simulink model "FULL_LINK"  (R2021b)
settings: Solver=VariableStepAuto  StartTime=0.0  StopTime=0.04  RelTol=1e-3
undefined symbols (not defined in the file): fcarrier
libraries: fl_lib x21, nesl_utility x7, dspsrcs4 x5, dspswit3 x4, ee_lib x3, dsparch4 x2, simulink x1, hdlsllib x1
settings Model: DataTypeOverride=Off  Creator=hp  LastModifiedBy=caccolillo
settings SolverCC: AlgebraicLoopSolver=TrustRegion  AutoInsertRateTranBlk=on
settings DataIOCC: ReturnWorkspaceOutputs=off
settings OptimizationCC: BlockReduction=off  ConditionallyExecuteInputs=off  DefaultParameterBehavior=Inlined  InheritOutputTypeSmallerThanSingle=on
settings DebuggingCC: AlgebraicLoopMsg=error  SingleTaskRateTransMsg=error  SFMachineParentedDataDiag=warning  ArithmeticOperatorsInVariantConditions=warning
settings HardwareCC: ProdBitPerPointer=32  ProdBitPerSizeT=32  ProdBitPerPtrDiffT=32  ProdLargestAtomicFloat=None  ProdIntDivRoundTo=Undefined  ProdEndianess=Unspecified  ProdWordSize=32  ProdHWDeviceType=ASIC/FPGA->ASIC/FPGA  TargetBitPerLong=64  TargetBitPerPointer=64  TargetBitPerSizeT=64  TargetBitPerPtrDiffT=64  TargetLongLongMode=on  TargetIntDivRoundTo=Zero  TargetEndianess=LittleEndian  TargetWordSize=64  TargetHWDeviceType=Custom Processor->MATLAB Host Computer  ProdEqTarget=off
settings SFSimCC: SimUseLocalCustomCode=off  CustomCodeUndefinedFunction=UseInterfaceOnly
settings RTWCC: RTWUseLocalCustomCode=off

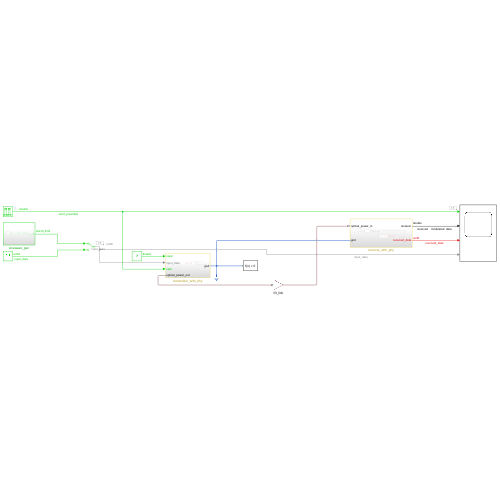
[thumbnail: Simulink's stored preview of the top-level diagram]
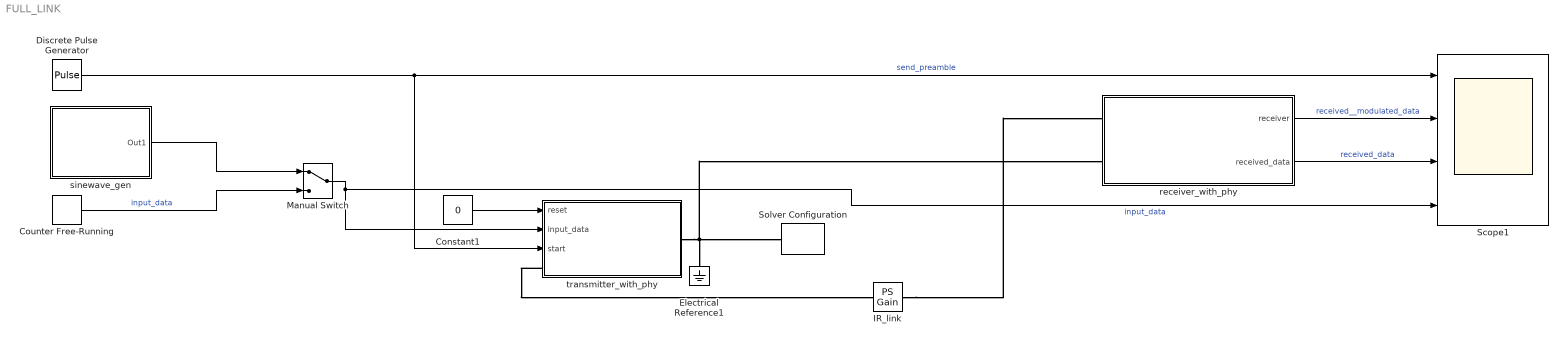
== system FULL_LINK ==
  Constant1 : Constant  Value=0  OutDataTypeStr=double  SampleTime=4/fcarrier
  Counter Free-Running : simulink/Sources/Counter Free-Running  NumBits=8  tsamp=4/fcarrier
  Discrete Pulse Generator : DiscretePulseGenerator  Period=20000  PhaseDelay=80  SampleTime=4/fcarrier
  Electrical Reference1 : fl_lib/Electrical/Electrical Elements/Electrical Reference
  IR_link : fl_lib/Physical Signals/Functions/PS Gain  gain=1e4 1/m^2
  Manual Switch : ManualSwitch
  Scope1 : Scope  NumInputPorts=4
  Solver Configuration : nesl_utility/Solver Configuration  PhysicalDomain=network_engine_domain  SubClassName=solver  LeftPortType=input  RightPortType=generic  Tones=[]  Harmonics=[]  SimulateNoise=off  Profile=off  UseLocalSampling=off  EnableSwitchedLinearOptims=on  FrequencyDomain=off  UseCCode=off  RelTol=0.001  AbsTol=1e-06  MinStep=1e-09  ToWorkspace=off  RevertToSquareIcSolve=off  NumHomotopyIterations=100  PhasorMode=off  PhasorModeNumHarmonics=1  DoDC=off  ResidualTolerance=1e-09  UseLocalSolver=off  LocalSolverChoice=NE_BACKWARD_EULER_ADVANCER  LocalSolverSampleTime=0.001  DoFixedCost=off  MaxNonlinIter=3  MaxModeIter=2  ComputeImpulses=off  ImpulseIterations=2  LinearAlgebra=auto  EquationFormulation=NE_TIME_EF  DelaysMemoryBudget=1024  AutomaticFiltering=on  FilteringTimeConstant=0.001  PartitionStorageMethod=AS_NEEDED  PartitionMemoryBudget=1024  PartitionMethod=ROBUST
      settings: SourceProductBaseCode=PW,SS
  receiver_with_phy : Subsystem
  sinewave_gen : Subsystem
  transmitter_with_phy : Subsystem
  wires:
  Discrete Pulse Generator/1 -> transmitter_with_phy/3(start), Scope1/1  "send_preamble"
  Manual Switch/1 -> transmitter_with_phy/2(input_data), Scope1/4  "input_data"
  Counter Free-Running/1 -> Manual Switch/2  "input_data"
  Constant1/1 -> transmitter_with_phy/1(reset)
  receiver_with_phy/2(received_data) -> Scope1/3  "received_data"
  receiver_with_phy/1(receiver) -> Scope1/2  "received__modulated_data"
  sinewave_gen/1(Out1) -> Manual Switch/1
  connections:
  transmitter_with_phy/RConn1 -- receiver_with_phy/LConn2 -- Solver Configuration/RConn1 -- Electrical Reference1/LConn1
  transmitter_with_phy/LConn1 -- IR_link/LConn1
  IR_link/RConn1 -- receiver_with_phy/LConn1

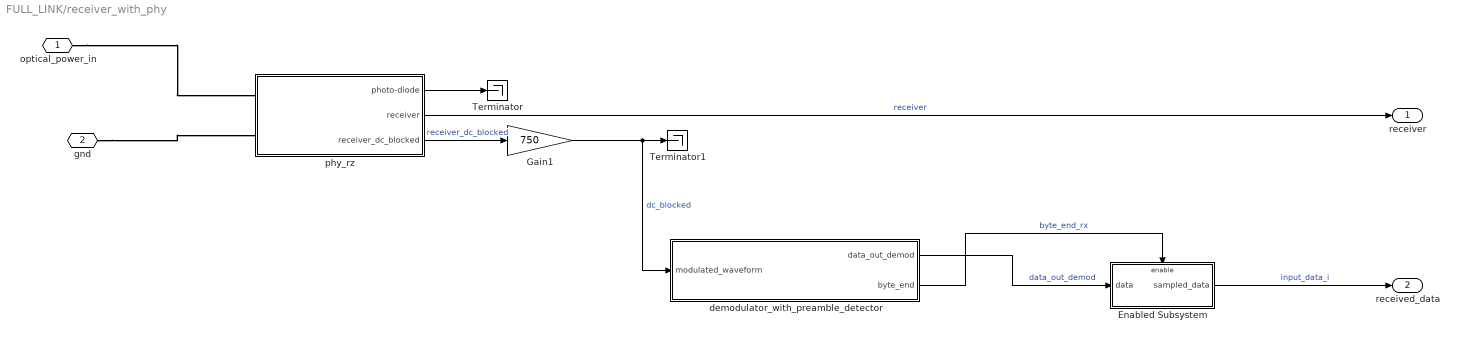
== system FULL_LINK/receiver_with_phy ==
  Enabled Subsystem : Subsystem  TreatAsAtomicUnit=on
  Gain1 : Gain  Gain=750
  Terminator : Terminator
  Terminator1 : Terminator
  demodulator_with_preamble_detector : Subsystem
  phy_rz : Subsystem
  optical_power_in : PMIOPort  Side=Left
  gnd : PMIOPort  Port=2  Side=Left
  receiver : Outport
  received_data : Outport  Port=2
  wires:
  phy_rz/3(receiver_dc_blocked) -> Gain1/1  "receiver_dc_blocked"
  phy_rz/1(photo-diode) -> Terminator/1
  Gain1/1 -> Terminator1/1, demodulator_with_preamble_detector/1(modulated_waveform)  "dc_blocked"
  demodulator_with_preamble_detector/2(byte_end) -> Enabled Subsystem/Enable  "byte_end_rx"
  phy_rz/2(receiver) -> receiver/1  "receiver"
  Enabled Subsystem/1(sampled_data) -> received_data/1  "input_data_i"
  demodulator_with_preamble_detector/1(data_out_demod) -> Enabled Subsystem/1(data)  "data_out_demod"
  connections:
  gnd/RConn1 -- phy_rz/LConn2
  optical_power_in/RConn1 -- phy_rz/LConn1

== system FULL_LINK/sinewave_gen ==
  Add Constant : Bias  Bias=128
  Data Type Conversion1 : DataTypeConversion  OutDataTypeStr=uint8
  Gain2 : Gain  Gain=1/4
  Sine Wave2 : dspsrcs4/Sine Wave  Amplitude=128  Frequency=fcarrier/150  Phase=0  SampleMode=Discrete  OutComplex=Real  CompMethod=Trigonometric fcn  TableSize=Speed  SampleTime=4/fcarrier  SamplesPerFrame=1  ResetState=Restart at time zero  OutputFrames=off  dataType=double  wordLen=16  udDataType=sfix(16)  fracBitsMode=Best precision  numFracBits=15  OutDataTypeStr=double  LastOutDataTypeStr=double
  Out1 : Outport
  wires:
  Sine Wave2/1 -> Data Type Conversion1/1
  Gain2/1 -> Out1/1
  Data Type Conversion1/1 -> Add Constant/1
  Add Constant/1 -> Gain2/1

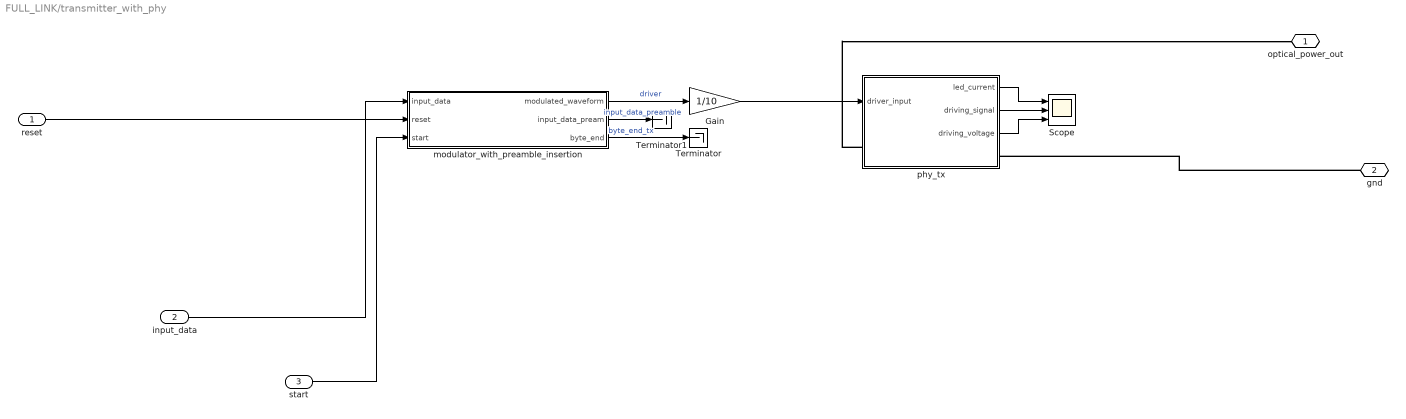
== system FULL_LINK/transmitter_with_phy ==
  reset : Inport
  input_data : Inport  Port=2
  start : Inport  Port=3
  Gain : Gain  Gain=1/10
  Scope : Scope  NumInputPorts=3
  Terminator : Terminator
  Terminator1 : Terminator
  modulator_with_preamble_insertion : Subsystem
  phy_tx : Subsystem
  optical_power_out : PMIOPort  Side=Left
  gnd : PMIOPort  Port=2  Side=Right
  wires:
  phy_tx/1(led_current) -> Scope/1
  Gain/1 -> phy_tx/1(driver_input)
  modulator_with_preamble_insertion/2(input_data_pream) -> Terminator1/1  "input_data_preamble"
  modulator_with_preamble_insertion/3(byte_end) -> Terminator/1  "byte_end_tx"
  start/1 -> modulator_with_preamble_insertion/3(start)
  phy_tx/2(driving_signal) -> Scope/2
  modulator_with_preamble_insertion/1(modulated_waveform) -> Gain/1  "driver"
  input_data/1 -> modulator_with_preamble_insertion/1(input_data)
  reset/1 -> modulator_with_preamble_insertion/2(reset)
  phy_tx/3(driving_voltage) -> Scope/3
  connections:
  gnd/RConn1 -- phy_tx/RConn1
  phy_tx/LConn1 -- optical_power_out/RConn1

== system FULL_LINK/receiver_with_phy/Enabled Subsystem ==
  data : Inport
  Enable : EnablePort
  sampled_data : Outport  InitialOutput=0
  wires:
  data/1 -> sampled_data/1

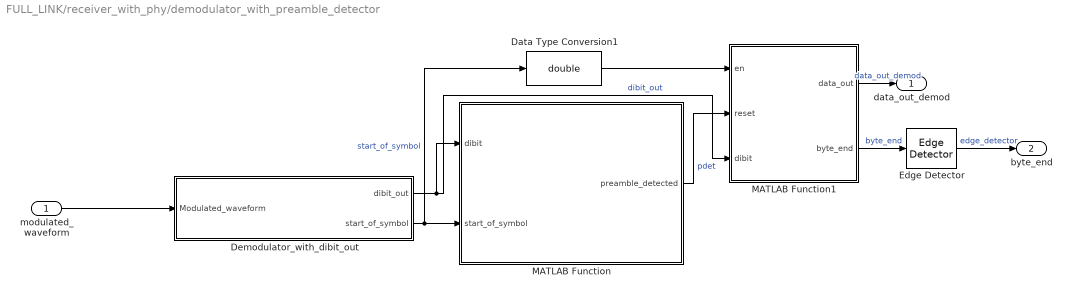
== system FULL_LINK/receiver_with_phy/demodulator_with_preamble_detector ==
  modulated_waveform : Inport
  Data Type Conversion1 : DataTypeConversion  OutDataTypeStr=double
  Demodulator_with_dibit_out : Subsystem
  Edge Detector : dspswit3/Edge Detector  InputProcessing=Columns as channels (frame based)
      settings: SourceProductBaseCode=DS
  MATLAB Function : MATLAB Function  TreatAsAtomicUnit=on
  MATLAB Function1 : MATLAB Function  TreatAsAtomicUnit=on
  data_out_demod : Outport
  byte_end : Outport  Port=2
  wires:
  Demodulator_with_dibit_out/1(dibit_out) -> MATLAB Function/1(dibit), MATLAB Function1/3(dibit)  "dibit_out"
  Demodulator_with_dibit_out/2(start_of_symbol) -> MATLAB Function/2(start_of_symbol), Data Type Conversion1/1  "start_of_symbol"
  Edge Detector/1 -> byte_end/1  "edge_detector"
  modulated_waveform/1 -> Demodulator_with_dibit_out/1(Modulated_waveform)
  MATLAB Function/1(preamble_detected) -> MATLAB Function1/2(reset)  "pdet"
  Data Type Conversion1/1 -> MATLAB Function1/1(en)
  MATLAB Function1/1(data_out) -> data_out_demod/1  "data_out_demod"
  MATLAB Function1/2(byte_end) -> Edge Detector/1  "byte_end"

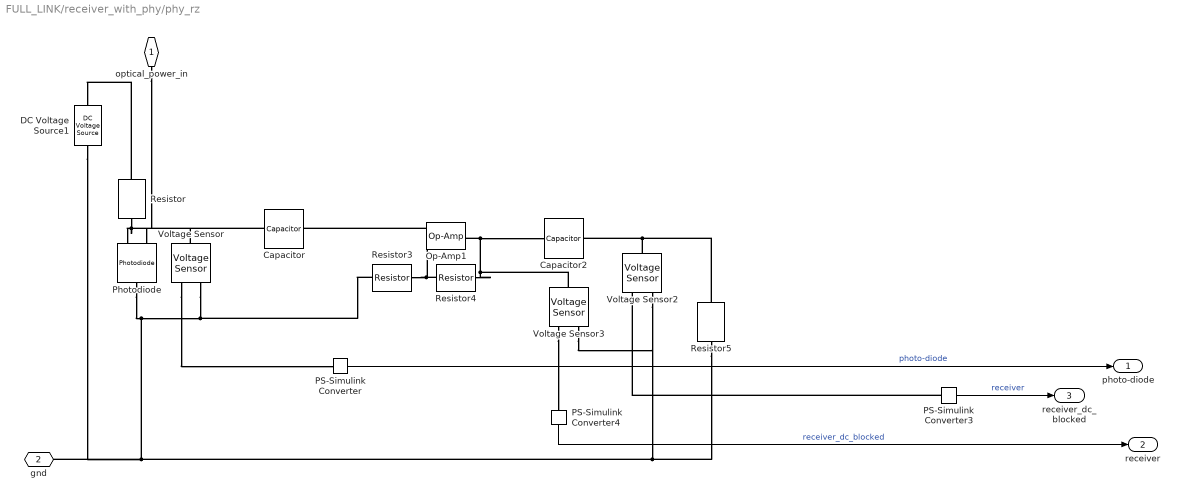
== system FULL_LINK/receiver_with_phy/phy_rz ==
  Capacitor : fl_lib/Electrical/Electrical Elements/Capacitor  c=10 uF  r=0 Ohm  g=0 1/Ohm  i_specify=off  i_priority=None  i=0 A  i_nominal_specify=off  i_nominal_unit=A  i_nominal_value=1  v_specify=off  v_priority=None  v=0 V  v_nominal_specify=off  v_nominal_unit=V  v_nominal_value=1  vc_specify=off  vc_priority=High  vc=0 V  vc_nominal_specify=off  vc_nominal_unit=V  vc_nominal_value=1
  Capacitor2 : fl_lib/Electrical/Electrical Elements/Capacitor  c=1 uF  r=0 Ohm  g=0 1/Ohm  i_specify=off  i_priority=None  i=0 A  i_nominal_specify=off  i_nominal_unit=A  i_nominal_value=1  v_specify=off  v_priority=None  v=0 V  v_nominal_specify=off  v_nominal_unit=V  v_nominal_value=1  vc_specify=off  vc_priority=High  vc=0 V  vc_nominal_specify=off  vc_nominal_unit=V  vc_nominal_value=1
  DC Voltage Source1 : fl_lib/Electrical/Electrical Sources/DC Voltage Source  v0=5 V
  Op-Amp1 : fl_lib/Electrical/Electrical Elements/Op-Amp  outI_specify=off  outI_priority=None  outI=0 A  outI_nominal_specify=off  outI_nominal_unit=A  outI_nominal_value=1
  PS-Simulink Converter : nesl_utility/PS-Simulink Converter  PhysicalDomain=network_engine_domain  SubClassName=ps_output  LeftPortType=input  RightPortType=output  PseudoPeriodic=off  Frequencies=[]  Unit=inherit  AffineConversion=off
      settings: SourceProductBaseCode=PW,SS
  PS-Simulink Converter3 : nesl_utility/PS-Simulink Converter  PhysicalDomain=network_engine_domain  SubClassName=ps_output  LeftPortType=input  RightPortType=output  PseudoPeriodic=off  Frequencies=[]  Unit=inherit  AffineConversion=off
      settings: SourceProductBaseCode=PW,SS
  PS-Simulink Converter4 : nesl_utility/PS-Simulink Converter  PhysicalDomain=network_engine_domain  SubClassName=ps_output  LeftPortType=input  RightPortType=output  PseudoPeriodic=off  Frequencies=[]  Unit=inherit  AffineConversion=off
      settings: SourceProductBaseCode=PW,SS
  Photodiode : ee_lib/Sensors & Transducers/Photodiode  prmFlux=1  Imeas=25 uA  FluxD=5 W/m^2  G=5e-6 A*m^2/W  prmExp=1  I2=0.1 A  V2=1.3 V  IS=5e-9 A  ec=3  RS=0.1 Ohm  Tmeas=25 degC  C_param=1  CJ=60 pF  CJ0=60 pF  VJ=1 V  Mgrad=0.5  Vvec=[.1, 10, 100] V  Cvec=[45, 3, 6] pF  FC=0.5  T_param=1  IS_T2=2.5e-7 A  I1_T2=0.07 A  V1_T2=1.3 V  Tmeas2=125 degC  EG_param=1  EG=1.11 eV  XTI_param=1  XTI=3  Tdevice=25 degC  i_capacitor_specify=off  i_capacitor_priority=High  i_capacitor=0 A  i_capacitor_nominal_specify=off  i_capacitor_nominal_unit=A  i_capacitor_nominal_value=1  v_capacitor_specify=off  v_capacitor_priority=None  v_capacitor=0 V  v_capacitor_nominal_specify=off  v_capacitor_nominal_unit=V  v_capacitor_nominal_value=1  thermal_network_parameterization=ee.enum.thermalNetworkTopology.junctionCase  Rth=[0, 10] K/W  Rth_Cauer=[1, 3, 10] K/W  Rth_Foster=[4, 6] K/W  thermal_mass_parameterization=ee.enum.thermalNetwork.timeconstant  thermal_mass=[0, 1] J/K  thermal_mass_Cauer=[1.5, 2, 3] J/K  thermal_mass_Foster=[1.5, 3] J/K  thermal_time_constant=[0, 10] s  thermal_time_constant_Cauer=[1, 3, 10] s  thermal_time_constant_Foster=[6, 18] s  thermal_mass_initial_temperatures=[25, 25] degC  thermal_mass_initial_temperatures_Cauer=[25, 25, 25] degC  steadyState_Foster=simscape.enum.onoff.on  Tvec_initial_Foster=[25, 25, 25, 25] degC
      settings: SourceProductBaseCode=PS  InternalSimscapePortConfiguration="{\"Bottom\":[],\"Left\":[{\"id\":\"W\",\"label\":\"W\",\"type\":\"input\"},{\"id\":\"p\",\"label\":\"\",\"type\":\"foundation.electrical.electrical\"}],\"Right\":[{\"id\":\"n\",\"label\":\"\",\"type\":\"foundation.electrical.electrical\"}],\"Top\":[]}"
  Resistor : fl_lib/Electrical/Electrical Elements/Resistor  R=1000 Ohm  i_specify=off  i_priority=None  i=0 A  i_nominal_specify=off  i_nominal_unit=A  i_nominal_value=1  v_specify=off  v_priority=None  v=0 V  v_nominal_specify=off  v_nominal_unit=V  v_nominal_value=1
  Resistor3 : fl_lib/Electrical/Electrical Elements/Resistor  R=1000 Ohm  i_specify=off  i_priority=None  i=0 A  i_nominal_specify=off  i_nominal_unit=A  i_nominal_value=1  v_specify=off  v_priority=None  v=0 V  v_nominal_specify=off  v_nominal_unit=V  v_nominal_value=1
  Resistor4 : fl_lib/Electrical/Electrical Elements/Resistor  R=20000 Ohm  i_specify=off  i_priority=None  i=0 A  i_nominal_specify=off  i_nominal_unit=A  i_nominal_value=1  v_specify=off  v_priority=None  v=0 V  v_nominal_specify=off  v_nominal_unit=V  v_nominal_value=1
  Resistor5 : fl_lib/Electrical/Electrical Elements/Resistor  R=1 kOhm  i_specify=off  i_priority=None  i=5 mA  i_nominal_specify=off  i_nominal_unit=A  i_nominal_value=1  v_specify=off  v_priority=None  v=0 V  v_nominal_specify=off  v_nominal_unit=V  v_nominal_value=1
  Voltage Sensor : fl_lib/Electrical/Electrical Sensors/Voltage Sensor
  Voltage Sensor2 : fl_lib/Electrical/Electrical Sensors/Voltage Sensor
  Voltage Sensor3 : fl_lib/Electrical/Electrical Sensors/Voltage Sensor
  optical_power_in : PMIOPort  Side=Left
  gnd : PMIOPort  Port=2  Side=Left
  photo-diode : Outport
  receiver : Outport  Port=2
  receiver_dc_blocked : Outport  Port=3
  wires:
  PS-Simulink Converter/1 -> photo-diode/1  "photo-diode"
  PS-Simulink Converter4/1 -> receiver/1  "receiver_dc_blocked"
  PS-Simulink Converter3/1 -> receiver_dc_blocked/1  "receiver"
  connections:
  PS-Simulink Converter3/LConn1 -- Voltage Sensor2/RConn1
  Resistor4/LConn1 -- Voltage Sensor3/LConn1 -- Capacitor2/LConn1 -- Op-Amp1/RConn1
  optical_power_in/RConn1 -- Photodiode/LConn1
  Resistor3/LConn1 -- Op-Amp1/LConn2 -- Resistor4/RConn1
  Op-Amp1/LConn1 -- Capacitor/RConn1
  Voltage Sensor3/RConn1 -- PS-Simulink Converter4/LConn1
  Resistor5/LConn1 -- Voltage Sensor2/RConn2 -- Voltage Sensor3/RConn2 -- Photodiode/RConn1 -- Resistor3/RConn1 -- Voltage Sensor/RConn2 -- DC Voltage Source1/RConn1 -- gnd/RConn1
  Voltage Sensor2/LConn1 -- Resistor5/RConn1 -- Capacitor2/RConn1
  Voltage Sensor/RConn1 -- PS-Simulink Converter/LConn1
  Resistor/LConn1 -- DC Voltage Source1/LConn1
  Resistor/RConn1 -- Voltage Sensor/LConn1 -- Capacitor/LConn1 -- Photodiode/LConn2

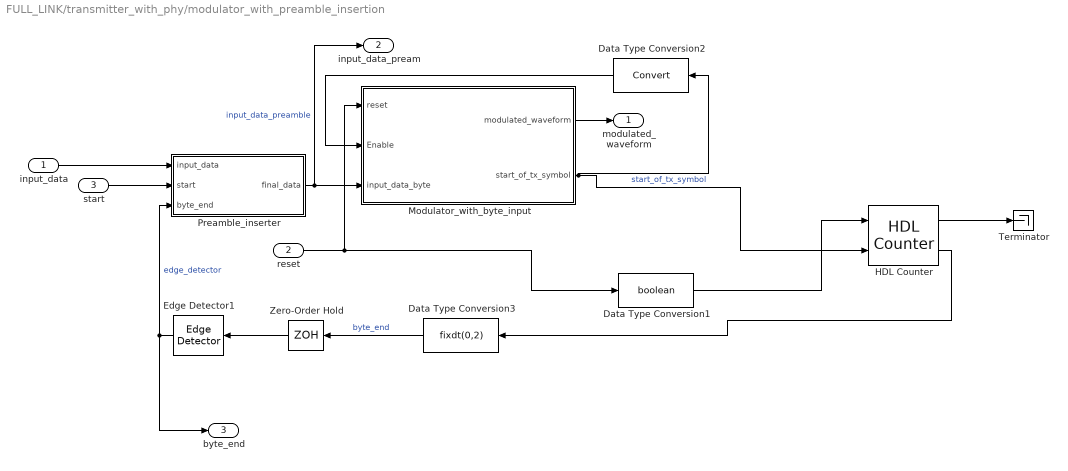
== system FULL_LINK/transmitter_with_phy/modulator_with_preamble_insertion ==
  input_data : Inport
  reset : Inport  Port=2
  start : Inport  Port=3
  Data Type Conversion1 : DataTypeConversion  OutDataTypeStr=boolean
  Data Type Conversion2 : DataTypeConversion
  Data Type Conversion3 : DataTypeConversion  OutMin=[0]  OutMax=[1]  OutDataTypeStr=fixdt(0,2)
  Edge Detector1 : dspswit3/Edge Detector  InputProcessing=Columns as channels (frame based)
      settings: SourceProductBaseCode=DS
  HDL Counter : hdlsllib/Sources/HDL Counter  CountType=Count limited  CountInit=0  CountStep=1  CountMax=7  CountFromType=Initial value  CountFrom=0  CountResetPort=on  CountLoadPort=off  CountEnbPort=on  CountDirPort=off  CountHitOutputPort=on  CountDataType=Unsigned  CountWordLen=8  CountFracLen=0  CountSampTime=1
  Modulator_with_byte_input : Subsystem
  Preamble_inserter : Subsystem
  Terminator : Terminator
  Zero-Order Hold : ZeroOrderHold  SampleTime=-1
  modulated_waveform : Outport
  input_data_pream : Outport  Port=2
  byte_end : Outport  Port=3
  wires:
  reset/1 -> Data Type Conversion1/1, Modulator_with_byte_input/1(reset)
  Modulator_with_byte_input/2(start_of_tx_symbol) -> HDL Counter/2, Data Type Conversion2/1  "start_of_tx_symbol"
  Data Type Conversion2/1 -> Modulator_with_byte_input/2(Enable)
  Modulator_with_byte_input/1(modulated_waveform) -> modulated_waveform/1
  Preamble_inserter/1(final_data) -> Modulator_with_byte_input/3(input_data_byte), input_data_pream/1  "input_data_preamble"
  Data Type Conversion3/1 -> Zero-Order Hold/1  "byte_end"
  HDL Counter/2 -> Data Type Conversion3/1
  start/1 -> Preamble_inserter/2(start)
  input_data/1 -> Preamble_inserter/1(input_data)
  Edge Detector1/1 -> byte_end/1, Preamble_inserter/3(byte_end)  "edge_detector"
  HDL Counter/1 -> Terminator/1
  Data Type Conversion1/1 -> HDL Counter/1
  Zero-Order Hold/1 -> Edge Detector1/1

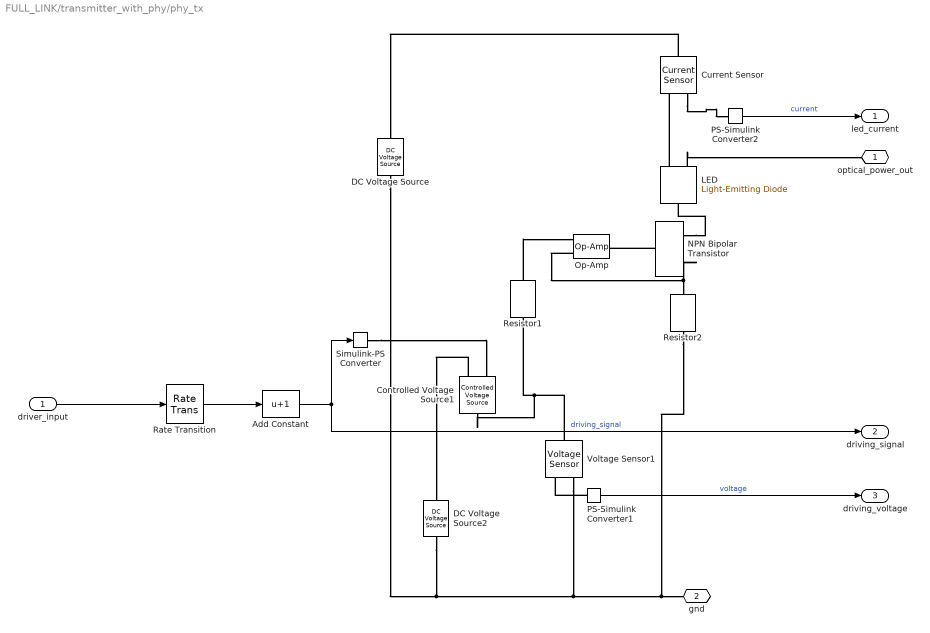
== system FULL_LINK/transmitter_with_phy/phy_tx ==
  driver_input : Inport
  Add Constant : Bias  Bias=1
  Controlled Voltage Source1 : fl_lib/Electrical/Electrical Sources/Controlled Voltage Source
  Current Sensor : fl_lib/Electrical/Electrical Sensors/Current Sensor
  DC Voltage Source : fl_lib/Electrical/Electrical Sources/DC Voltage Source  v0=3 V
  DC Voltage Source2 : fl_lib/Electrical/Electrical Sources/DC Voltage Source  v0=0.1 V
  LED : ee_lib/Sensors & Transducers/Light-Emitting Diode  Gain=0.005 W/A  prmExp=1  I12=[.0017, .003] A  V12=[.9, 1.05] V  IS=5e-5 A  ec=10  RS=0.1 Ohm  Tmeas=25 degC  C_param=1  CJ=20 pF  CJ0=20 pF  VJ=1 V  Mgrad=0.5  Vvec=[.1, 10, 100] V  Cvec=[15, 10, 2] pF  FC=0.5  T_param=1  IS_T2=1.8e-4 A  I1_T2=0.0034 A  V1_T2=1.05 V  Tmeas2=125 degC  EG_param=1  EG=1.11 eV  XTI_param=1  XTI=3  Tdevice=25 degC  i_capacitor_specify=off  i_capacitor_priority=High  i_capacitor=0 A  i_capacitor_nominal_specify=off  i_capacitor_nominal_unit=A  i_capacitor_nominal_value=1  v_capacitor_specify=off  v_capacitor_priority=None  v_capacitor=0 V  v_capacitor_nominal_specify=off  v_capacitor_nominal_unit=V  v_capacitor_nominal_value=1  thermal_network_parameterization=ee.enum.thermalNetworkTopology.junctionCase  Rth=[0, 10] K/W  Rth_Cauer=[1, 3, 10] K/W  Rth_Foster=[4, 6] K/W  thermal_mass_parameterization=ee.enum.thermalNetwork.timeconstant  thermal_mass=[0, 1] J/K  thermal_mass_Cauer=[1.5, 2, 3] J/K  thermal_mass_Foster=[1.5, 3] J/K  thermal_time_constant=[0, 10] s  thermal_time_constant_Cauer=[1, 3, 10] s  thermal_time_constant_Foster=[6, 18] s  thermal_mass_initial_temperatures=[25, 25] degC  thermal_mass_initial_temperatures_Cauer=[25, 25, 25] degC  steadyState_Foster=simscape.enum.onoff.on  Tvec_initial_Foster=[25, 25, 25, 25] degC
      settings: SourceProductBaseCode=PS  InternalSimscapePortConfiguration="{\"Bottom\":[],\"Left\":[{\"id\":\"W\",\"label\":\"W\",\"type\":\"output\"},{\"id\":\"p\",\"label\":\"\",\"type\":\"foundation.electrical.electrical\"}],\"Right\":[{\"id\":\"n\",\"label\":\"\",\"type\":\"foundation.electrical.electrical\"}],\"Top\":[]}"
  NPN Bipolar Transistor : ee_lib/Semiconductors & Converters/NPN Bipolar Transistor  parameterization=1  BF=100  IS=1e-14 A  VAF=200 V  hfe=100  hoe=50e-6 1/Ohm  Ic_h=1 mA  Vce_h=5 V  V1=0.55 V  I1=0.5 mA  BR=1  Tmeas=25 degC  RC=0.01 Ohm  RE=1e-4 Ohm  RB=1 Ohm  C_BC=5 pF  C_BE=5 pF  TF=0 us  TR=0 us  prmDatasheet=1  prmEquCoeff=1  hfe_T2=125  XTB=0  V1_T2=0.45 V  I1_T2=0.5 mA  Tmeas2=125 degC  EG=1.11 eV  XTI=3  TdeviceDatasheet=25 degC  TdeviceEquCoeff=25 degC  ec=1  thermal_network_parameterization=ee.enum.thermalNetworkTopology.junctionCase  Rth=[0, 10] K/W  Rth_Cauer=[1, 3, 10] K/W  Rth_Foster=[4, 6] K/W  thermal_mass_parameterization=ee.enum.thermalNetwork.timeconstant  thermal_mass=[0, 1] J/K  thermal_mass_Cauer=[.1, .3, 1] J/K  thermal_mass_Foster=[1.5, 3] J/K  thermal_time_constant=[0, 10] s  thermal_time_constant_Cauer=[1, 3, 10] s  thermal_time_constant_Foster=[6, 18] s  thermal_mass_initial_temperatures=[25, 25] degC  thermal_mass_initial_temperatures_Cauer=[25, 25, 25] degC  steadyState_Foster=simscape.enum.onoff.on  Tvec_initial_Foster=[25, 25, 25, 25] degC
  Op-Amp : fl_lib/Electrical/Electrical Elements/Op-Amp  outI_specify=off  outI_priority=None  outI=0 A  outI_nominal_specify=off  outI_nominal_unit=A  outI_nominal_value=1
  PS-Simulink Converter1 : nesl_utility/PS-Simulink Converter  PhysicalDomain=network_engine_domain  SubClassName=ps_output  LeftPortType=input  RightPortType=output  PseudoPeriodic=off  Frequencies=[]  Unit=inherit  AffineConversion=off
      settings: SourceProductBaseCode=PW,SS
  PS-Simulink Converter2 : nesl_utility/PS-Simulink Converter  PhysicalDomain=network_engine_domain  SubClassName=ps_output  LeftPortType=input  RightPortType=output  PseudoPeriodic=off  Frequencies=[]  Unit=inherit  AffineConversion=off
      settings: SourceProductBaseCode=PW,SS
  Rate Transition : RateTransition
  Resistor1 : fl_lib/Electrical/Electrical Elements/Resistor  R=500 Ohm  i_specify=off  i_priority=None  i=0 A  i_nominal_specify=off  i_nominal_unit=A  i_nominal_value=1  v_specify=off  v_priority=None  v=0 V  v_nominal_specify=off  v_nominal_unit=V  v_nominal_value=1
  Resistor2 : fl_lib/Electrical/Electrical Elements/Resistor  R=10 Ohm  i_specify=off  i_priority=None  i=0 A  i_nominal_specify=off  i_nominal_unit=A  i_nominal_value=1  v_specify=off  v_priority=None  v=0 V  v_nominal_specify=off  v_nominal_unit=V  v_nominal_value=1
  Simulink-PS Converter : nesl_utility/Simulink-PS Converter  PhysicalDomain=network_engine_domain  SubClassName=ps_input  LeftPortType=input  RightPortType=output  PseudoPeriodic=off  Frequencies=[]  NoiseDistribution=none  NoiseParameters=[]  Unit=1  AffineConversion=off  FilteringAndDerivatives=provide  SimscapeFilterOrder=1  InputFilterTimeConstant=0.001  UdotUserProvided=0
      settings: SourceProductBaseCode=PW,SS
  Voltage Sensor1 : fl_lib/Electrical/Electrical Sensors/Voltage Sensor
  optical_power_out : PMIOPort  Side=Left
  gnd : PMIOPort  Port=2  Side=Right
  led_current : Outport
  driving_signal : Outport  Port=2
  driving_voltage : Outport  Port=3
  wires:
  PS-Simulink Converter2/1 -> led_current/1  "current"
  PS-Simulink Converter1/1 -> driving_voltage/1  "voltage"
  Add Constant/1 -> driving_signal/1, Simulink-PS Converter/1  "driving_signal"
  driver_input/1 -> Rate Transition/1
  Rate Transition/1 -> Add Constant/1
  connections:
  Controlled Voltage Source1/RConn2 -- DC Voltage Source2/LConn1
  Resistor1/RConn1 -- Op-Amp/LConn1
  Current Sensor/LConn1 -- DC Voltage Source/LConn1
  LED/LConn1 -- optical_power_out/RConn1
  Simulink-PS Converter/RConn1 -- Controlled Voltage Source1/RConn1
  DC Voltage Source2/RConn1 -- gnd/RConn1 -- Resistor2/RConn1 -- Voltage Sensor1/RConn2 -- DC Voltage Source/RConn1
  Current Sensor/RConn1 -- PS-Simulink Converter2/LConn1
  NPN Bipolar Transistor/RConn2 -- Op-Amp/LConn2 -- Resistor2/LConn1
  NPN Bipolar Transistor/LConn1 -- Op-Amp/RConn1
  NPN Bipolar Transistor/RConn1 -- LED/RConn1
  PS-Simulink Converter1/LConn1 -- Voltage Sensor1/RConn1
  Controlled Voltage Source1/LConn1 -- Voltage Sensor1/LConn1 -- Resistor1/LConn1
  LED/LConn2 -- Current Sensor/RConn2

== system FULL_LINK/receiver_with_phy/demodulator_with_preamble_detector/Demodulator_with_dibit_out ==
  Modulated_waveform : Inport
  Convert_to_decimal : Subsystem
  Demodulator_with_output_register : Subsystem
  dibit_out : Outport
  start_of_symbol : Outport  Port=2
  wires:
  Demodulator_with_output_register/1(i_demod) -> Convert_to_decimal/2(bit1)
  Demodulator_with_output_register/2(q_demod) -> Convert_to_decimal/1(bit0)
  Convert_to_decimal/1(convert) -> dibit_out/1  "dibit_out"
  Demodulator_with_output_register/3(start_of_symbol) -> start_of_symbol/1
  Modulated_waveform/1 -> Demodulator_with_output_register/1(Modulated_waveform)

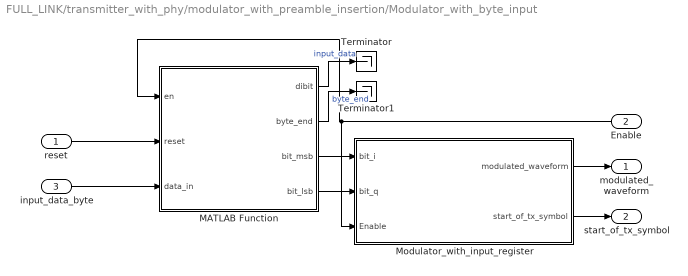
== system FULL_LINK/transmitter_with_phy/modulator_with_preamble_insertion/Modulator_with_byte_input ==
  reset : Inport
  Enable : Inport  Port=2
  input_data_byte : Inport  Port=3
  MATLAB Function : MATLAB Function  TreatAsAtomicUnit=on
  Modulator_with_input_register : Subsystem
  Terminator : Terminator
  Terminator1 : Terminator
  modulated_waveform : Outport
  start_of_tx_symbol : Outport  Port=2
  wires:
  Enable/1 -> MATLAB Function/1(en), Modulator_with_input_register/3(Enable)
  MATLAB Function/2(byte_end) -> Terminator1/1  "byte_end"
  Modulator_with_input_register/2(start_of_tx_symbol) -> start_of_tx_symbol/1
  input_data_byte/1 -> MATLAB Function/3(data_in)
  reset/1 -> MATLAB Function/2(reset)
  MATLAB Function/1(dibit) -> Terminator/1  "input_data"
  MATLAB Function/4(bit_lsb) -> Modulator_with_input_register/2(bit_q)
  Modulator_with_input_register/1(modulated_waveform) -> modulated_waveform/1
  MATLAB Function/3(bit_msb) -> Modulator_with_input_register/1(bit_i)

== system FULL_LINK/transmitter_with_phy/modulator_with_preamble_insertion/Preamble_inserter ==
  input_data : Inport
  start : Inport  Port=2
  byte_end : Inport  Port=3
  Chart : Stateflow chart  TreatAsAtomicUnit=on
      settings: PortSchema="{\"entries\":[{\"content\":{\"sides\":[{\"content\":{\"connectorIds\":[\"In2\"]},\"type\":\"ConnectorPlacement.EquallySpacedRectSide\",\"uuid\":\"c7ea0b9c-d106-4bd1-82e3-4c4e9722273c\"},{\"content\":{\"connectorIds\":[\"Out1\",\"Out2\"],\"side\":\"RIGHT\"},\"type\":\"ConnectorPlacement.EquallySpacedRectSide\",\"uuid\":\"4cc951b6-537b-4e23-ae77-107cf1cb9d20\"},{\"content\":{\"connectorIds\":[\"In1\"],\"side\":\"TOP\"},\"type\":\"ConnectorPlacement.EquallySpacedRectSide\",\"uuid\":\"96187a88-f84a-4d19-a7a7-49870645ca9d\"}]},\"type\":\"ConnectorPlacement.EquallySpacedConnector\",\"uuid\":\"a478a027-a6f7-4a96-ae1b-a22c0dc62afa\"}],\"packageUris\":[\"http://schema.mathworks.com/mf0/Connector/R2020b\"],\"version\":\"1.0\"}"
  Data Type Conversion4 : DataTypeConversion  OutMin=[0]  OutMax=[1]  OutDataTypeStr=double
  Switch : Switch  Criteria=u2 ~= 0  Threshold=1
  final_data : Outport
  wires:
  Switch/1 -> final_data/1  "final_data"
  input_data/1 -> Switch/1
  Data Type Conversion4/1 -> Switch/3
  Chart/2(select_data_preamble) -> Switch/2  "select_data_preamble"
  byte_end/1 -> Chart/1(byte_end)  "byte_end"
  Chart/1(input_data_byte) -> Data Type Conversion4/1  "input_data_byte"
  start/1 -> Chart/2(start)

== system FULL_LINK/receiver_with_phy/demodulator_with_preamble_detector/Demodulator_with_dibit_out/Convert_to_decimal ==
  bit0 : Inport
  bit1 : Inport  Port=2
  Add : Sum
  Gain1 : Gain  Gain=2
  convert : Outport
  wires:
  bit1/1 -> Gain1/1
  bit0/1 -> Add/1
  Add/1 -> convert/1  "convert"
  Gain1/1 -> Add/2

== system FULL_LINK/receiver_with_phy/demodulator_with_preamble_detector/Demodulator_with_dibit_out/Demodulator_with_output_register ==
  Modulated_waveform : Inport
  Demodulator : Subsystem
  Enabled Subsystem2 : Subsystem  TreatAsAtomicUnit=on
  Enabled Subsystem3 : Subsystem  TreatAsAtomicUnit=on
  i_demod : Outport
  q_demod : Outport  Port=2
  start_of_symbol : Outport  Port=3
  wires:
  Demodulator/2(q_demodulator) -> Enabled Subsystem3/1(bit_msb)  "q_demod"
  Demodulator/3(start_of_symbol) -> start_of_symbol/1, Enabled Subsystem3/Enable, Enabled Subsystem2/Enable
  Modulated_waveform/1 -> Demodulator/1(Modulated_waveform)
  Demodulator/1(i_demodulator) -> Enabled Subsystem2/1(bit_msb)  "i_demod"
  Enabled Subsystem2/1(i_data) -> i_demod/1  "i_demod"
  Enabled Subsystem3/1(i_data) -> q_demod/1  "q_demod"

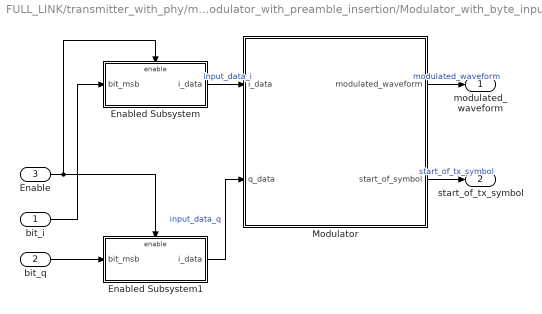
== system FULL_LINK/transmitter_with_phy/modulator_with_preamble_insertion/Modulator_with_byte_input/Modulator_with_input_register ==
  bit_i : Inport
  bit_q : Inport  Port=2
  Enable : Inport  Port=3
  Enabled Subsystem : Subsystem  TreatAsAtomicUnit=on
  Enabled Subsystem1 : Subsystem  TreatAsAtomicUnit=on
  Modulator : Subsystem
  modulated_waveform : Outport
  start_of_tx_symbol : Outport  Port=2
  wires:
  Enabled Subsystem/1(i_data) -> Modulator/1(i_data)  "input_data_i"
  Modulator/2(start_of_symbol) -> start_of_tx_symbol/1  "start_of_tx_symbol"
  bit_q/1 -> Enabled Subsystem1/1(bit_msb)
  bit_i/1 -> Enabled Subsystem/1(bit_msb)
  Enabled Subsystem1/1(i_data) -> Modulator/2(q_data)  "input_data_q"
  Modulator/1(modulated_waveform) -> modulated_waveform/1  "modulated_waveform"
  Enable/1 -> Enabled Subsystem/Enable, Enabled Subsystem1/Enable

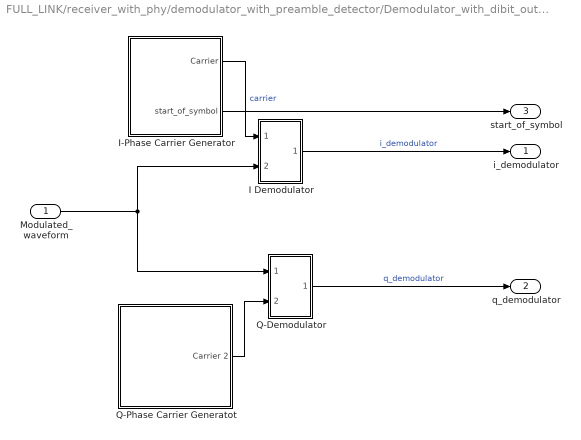
== system FULL_LINK/receiver_with_phy/demodulator_with_preamble_detector/Demodulator_with_dibit_out/Demodulator_with_output_register/Demodulator ==
  Modulated_waveform : Inport
  "I Demodulator " : Subsystem
  "I-Phase Carrier Generator " : Subsystem
  Q-Demodulator : Subsystem
  Q-Phase Carrier Generatot : Subsystem
  i_demodulator : Outport
  q_demodulator : Outport  Port=2
  start_of_symbol : Outport  Port=3
  wires:
  Q-Demodulator/1(Out1) -> q_demodulator/1  "q_demodulator"
  Modulated_waveform/1 -> Q-Demodulator/1(In1), "I Demodulator "/2(In2)
  Q-Phase Carrier Generatot/1("Carrier 2 ") -> Q-Demodulator/2("Carrier 2 ")
  "I Demodulator "/1(Out1) -> i_demodulator/1  "i_demodulator"
  "I-Phase Carrier Generator "/1(Carrier) -> "I Demodulator "/1(Carrier)  "carrier"
  "I-Phase Carrier Generator "/2(start_of_symbol) -> start_of_symbol/1

== system FULL_LINK/receiver_with_phy/demodulator_with_preamble_detector/Demodulator_with_dibit_out/Demodulator_with_output_register/Enabled Subsystem2 ==
  bit_msb : Inport
  Enable : EnablePort
  i_data : Outport  InitialOutput=0
  wires:
  bit_msb/1 -> i_data/1

== system FULL_LINK/receiver_with_phy/demodulator_with_preamble_detector/Demodulator_with_dibit_out/Demodulator_with_output_register/Enabled Subsystem3 ==
  bit_msb : Inport
  Enable : EnablePort
  i_data : Outport  InitialOutput=0
  wires:
  bit_msb/1 -> i_data/1

== system FULL_LINK/transmitter_with_phy/modulator_with_preamble_insertion/Modulator_with_byte_input/Modulator_with_input_register/Enabled Subsystem ==
  bit_msb : Inport
  Enable : EnablePort
  i_data : Outport  InitialOutput=0
  wires:
  bit_msb/1 -> i_data/1

== system FULL_LINK/transmitter_with_phy/modulator_with_preamble_insertion/Modulator_with_byte_input/Modulator_with_input_register/Enabled Subsystem1 ==
  bit_msb : Inport
  Enable : EnablePort
  i_data : Outport  InitialOutput=0
  wires:
  bit_msb/1 -> i_data/1

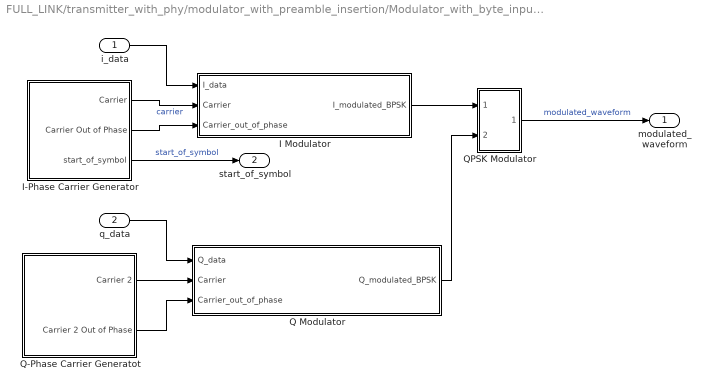
== system FULL_LINK/transmitter_with_phy/modulator_with_preamble_insertion/Modulator_with_byte_input/Modulator_with_input_register/Modulator ==
  i_data : Inport
  q_data : Inport  Port=2
  I Modulator : Subsystem
  "I-Phase Carrier Generator " : Subsystem
  Q Modulator : Subsystem
  Q-Phase Carrier Generatot : Subsystem
  QPSK Modulator : Subsystem
  modulated_waveform : Outport
  start_of_symbol : Outport  Port=2
  wires:
  I Modulator/1(I_modulated_BPSK) -> QPSK Modulator/1(In1)
  q_data/1 -> Q Modulator/1(Q_data)
  i_data/1 -> I Modulator/1(I_data)
  Q Modulator/1("Q_modulated_BPSK ") -> QPSK Modulator/2(In2)
  QPSK Modulator/1(Out1) -> modulated_waveform/1  "modulated_waveform"
  "I-Phase Carrier Generator "/2("Carrier Out of Phase ") -> I Modulator/3(Carrier_out_of_phase)
  Q-Phase Carrier Generatot/1("Carrier 2 ") -> Q Modulator/2(Carrier)
  Q-Phase Carrier Generatot/2(Carrier 2 Out of Phase) -> Q Modulator/3(Carrier_out_of_phase)
  "I-Phase Carrier Generator "/1(Carrier) -> I Modulator/2(Carrier)  "carrier"
  "I-Phase Carrier Generator "/3(start_of_symbol) -> start_of_symbol/1  "start_of_symbol"

== system FULL_LINK/receiver_with_phy/demodulator_with_preamble_detector/Demodulator_with_dibit_out/Demodulator_with_output_register/Demodulator/I Demodulator  ==
  Carrier : Inport
  In2 : Inport  Port=2
  Digital Filter Design : dsparch4/Digital Filter Design  mwdsp_browser_bugfix_var=off
  Product2 : Product
  Relational Operator : RelationalOperator  Operator=<  OutDataTypeStr=boolean  RndMeth=Simplest
  Scope : Scope  NumInputPorts=3
  Zero : Constant  Value=0  SampleTime=1/(100*fcarrier)
  Out1 : Outport  VectorParamsAs1DForOutWhenUnconnected=off
  wires:
  Digital Filter Design/1 -> Scope/3, Relational Operator/1  "filter_out"
  In2/1 -> Product2/2
  Product2/1 -> Scope/2, Digital Filter Design/1  "mixed"
  Zero/1 -> Relational Operator/2
  Relational Operator/1 -> Out1/1
  Carrier/1 -> Scope/1, Product2/1

== system FULL_LINK/receiver_with_phy/demodulator_with_preamble_detector/Demodulator_with_dibit_out/Demodulator_with_output_register/Demodulator/I-Phase Carrier Generator  ==
  Constant1 : Constant  Value=0  OutDataTypeStr=int8  SampleTime=1/(100*fcarrier)
  Data Type Conversion : DataTypeConversion  OutDataTypeStr=int8
  Edge Detector : dspswit3/Edge Detector  InputProcessing=Columns as channels (frame based)
      settings: SourceProductBaseCode=DS
  Equal : RelationalOperator  Operator=>  OutDataTypeStr=boolean  RndMeth=Simplest
  Scope : Scope  NumInputPorts=4
  Sine Wave1 : dspsrcs4/Sine Wave  Amplitude=1  Frequency=fcarrier  Phase=0  SampleMode=Discrete  OutComplex=Real  CompMethod=Trigonometric fcn  TableSize=Speed  SampleTime=1/(100*fcarrier)  SamplesPerFrame=1  ResetState=Restart at time zero  OutputFrames=off  dataType=double  wordLen=16  udDataType=sfix(16)  fracBitsMode=Best precision  numFracBits=15  OutDataTypeStr=double  LastOutDataTypeStr=double
  Carrier : Outport  VectorParamsAs1DForOutWhenUnconnected=off
  start_of_symbol : Outport  Port=2
  wires:
  Constant1/1 -> Equal/1
  Equal/1 -> Scope/2, Edge Detector/1  "start_of_symbol"
  Data Type Conversion/1 -> Scope/1, Equal/2
  Edge Detector/1 -> Scope/4, start_of_symbol/1  "edge_detector"
  Sine Wave1/1 -> Data Type Conversion/1, Scope/3, Carrier/1  "sine"

== system FULL_LINK/receiver_with_phy/demodulator_with_preamble_detector/Demodulator_with_dibit_out/Demodulator_with_output_register/Demodulator/Q-Demodulator ==
  In1 : Inport
  "Carrier 2 " : Inport  Port=2
  Digital Filter Design1 : dsparch4/Digital Filter Design  mwdsp_browser_bugfix_var=off
  Product3 : Product
  Relational Operator1 : RelationalOperator  Operator=<  OutDataTypeStr=boolean  RndMeth=Simplest
  Zero1 : Constant  Value=0  SampleTime=1/(100*fcarrier)
  Out1 : Outport  VectorParamsAs1DForOutWhenUnconnected=off
  wires:
  Zero1/1 -> Relational Operator1/2
  Digital Filter Design1/1 -> Relational Operator1/1
  Product3/1 -> Digital Filter Design1/1
  "Carrier 2 "/1 -> Product3/1
  Relational Operator1/1 -> Out1/1
  In1/1 -> Product3/2

== system FULL_LINK/receiver_with_phy/demodulator_with_preamble_detector/Demodulator_with_dibit_out/Demodulator_with_output_register/Demodulator/Q-Phase Carrier Generatot ==
  Sine Wave2 : dspsrcs4/Sine Wave  Amplitude=1  Frequency=fcarrier  Phase=pi/2  SampleMode=Discrete  OutComplex=Real  CompMethod=Trigonometric fcn  TableSize=Speed  SampleTime=1/(100*fcarrier)  SamplesPerFrame=1  ResetState=Restart at time zero  OutputFrames=off  dataType=double  wordLen=16  udDataType=sfix(16)  fracBitsMode=Best precision  numFracBits=15  OutDataTypeStr=double  LastOutDataTypeStr=double
  "Carrier 2 " : Outport  VectorParamsAs1DForOutWhenUnconnected=off
  wires:
  Sine Wave2/1 -> "Carrier 2 "/1

== system FULL_LINK/transmitter_with_phy/modulator_with_preamble_insertion/Modulator_with_byte_input/Modulator_with_input_register/Modulator/I Modulator ==
  I_data : Inport
  Carrier : Inport  Port=2
  Carrier_out_of_phase : Inport  Port=3
  Switch : Switch  Criteria=u2 > Threshold  Threshold=0.5
  I_modulated_BPSK : Outport  VectorParamsAs1DForOutWhenUnconnected=off
  wires:
  Carrier/1 -> Switch/3
  Carrier_out_of_phase/1 -> Switch/1
  I_data/1 -> Switch/2
  Switch/1 -> I_modulated_BPSK/1

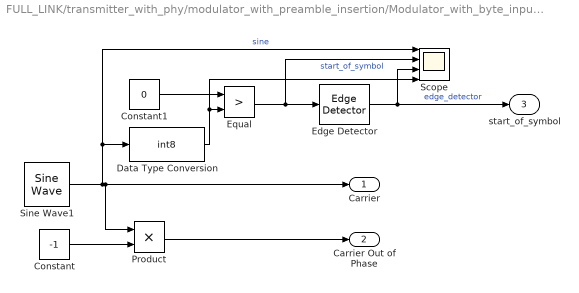
== system FULL_LINK/transmitter_with_phy/modulator_with_preamble_insertion/Modulator_with_byte_input/Modulator_with_input_register/Modulator/I-Phase Carrier Generator  ==
  Constant : Constant  Value=-1  SampleTime=1/(100*fcarrier)
  Constant1 : Constant  Value=0  OutDataTypeStr=int8  SampleTime=1/(100*fcarrier)
  Data Type Conversion : DataTypeConversion  OutDataTypeStr=int8  SaturateOnIntegerOverflow=on
  Edge Detector : dspswit3/Edge Detector  InputProcessing=Columns as channels (frame based)
      settings: SourceProductBaseCode=DS
  Equal : RelationalOperator  Operator=>  OutDataTypeStr=boolean  RndMeth=Simplest
  Product : Product
  Scope : Scope  NumInputPorts=4
  Sine Wave1 : dspsrcs4/Sine Wave  Amplitude=1  Frequency=fcarrier  Phase=0  SampleMode=Discrete  OutComplex=Real  CompMethod=Trigonometric fcn  TableSize=Speed  SampleTime=1/(100*fcarrier)  SamplesPerFrame=1  ResetState=Restart at time zero  OutputFrames=off  dataType=double  wordLen=16  udDataType=sfix(16)  fracBitsMode=Best precision  numFracBits=15  OutDataTypeStr=double  LastOutDataTypeStr=double
  Carrier : Outport  VectorParamsAs1DForOutWhenUnconnected=off
  "Carrier Out of Phase " : Outport  Port=2  VectorParamsAs1DForOutWhenUnconnected=off
  start_of_symbol : Outport  Port=3
  wires:
  Constant/1 -> Product/2
  Product/1 -> "Carrier Out of Phase "/1
  Sine Wave1/1 -> Carrier/1, Product/1, Scope/1, Data Type Conversion/1  "sine"
  Equal/1 -> Scope/2, Edge Detector/1  "start_of_symbol"
  Constant1/1 -> Equal/1
  Data Type Conversion/1 -> Scope/4, Equal/2
  Edge Detector/1 -> Scope/3, start_of_symbol/1  "edge_detector"

== system FULL_LINK/transmitter_with_phy/modulator_with_preamble_insertion/Modulator_with_byte_input/Modulator_with_input_register/Modulator/Q Modulator ==
  Q_data : Inport
  Carrier : Inport  Port=2
  Carrier_out_of_phase : Inport  Port=3
  Switch1 : Switch  Criteria=u2 > Threshold  Threshold=0.5
  "Q_modulated_BPSK " : Outport  VectorParamsAs1DForOutWhenUnconnected=off
  wires:
  Q_data/1 -> Switch1/2
  Carrier_out_of_phase/1 -> Switch1/1
  Switch1/1 -> "Q_modulated_BPSK "/1
  Carrier/1 -> Switch1/3

== system FULL_LINK/transmitter_with_phy/modulator_with_preamble_insertion/Modulator_with_byte_input/Modulator_with_input_register/Modulator/Q-Phase Carrier Generatot ==
  Constant1 : Constant  Value=-1  SampleTime=1/(100*fcarrier)
  Product1 : Product
  Sine Wave2 : dspsrcs4/Sine Wave  Amplitude=1  Frequency=fcarrier  Phase=pi/2  SampleMode=Discrete  OutComplex=Real  CompMethod=Trigonometric fcn  TableSize=Speed  SampleTime=1/(100*fcarrier)  SamplesPerFrame=1  ResetState=Restart at time zero  OutputFrames=off  dataType=double  wordLen=16  udDataType=sfix(16)  fracBitsMode=Best precision  numFracBits=15  OutDataTypeStr=double  LastOutDataTypeStr=double
  "Carrier 2 " : Outport  VectorParamsAs1DForOutWhenUnconnected=off
  Carrier 2 Out of Phase : Outport  Port=2  VectorParamsAs1DForOutWhenUnconnected=off
  wires:
  Constant1/1 -> Product1/2
  Sine Wave2/1 -> Product1/1, "Carrier 2 "/1
  Product1/1 -> Carrier 2 Out of Phase/1

== system FULL_LINK/transmitter_with_phy/modulator_with_preamble_insertion/Modulator_with_byte_input/Modulator_with_input_register/Modulator/QPSK Modulator ==
  In1 : Inport
  In2 : Inport  Port=2
  Add : Sum
  Out1 : Outport  VectorParamsAs1DForOutWhenUnconnected=off
  wires:
  In2/1 -> Add/2
  In1/1 -> Add/1
  Add/1 -> Out1/1

== matlab function FULL_LINK/receiver_with_phy/demodulator_with_preamble_detector/MATLAB Function ==
  settings: fimath=fimath('RoundingMethod', 'Floor','OverflowAction', 'Wrap','ProductMode', 'FullPrecision', 'SumMode', 'FullPrecision')
  data: dibit input; preamble_detected output; start_of_symbol input
function preamble_detected = detect_preamble(dibit, start_of_symbol)
%DETECT_PREAMBLE Detects a run of at least 31 consecutive dibit==2,
%followed by dibit==3 (only evaluated when start_of_symbol == 1).
%
% State Machine:
%   State 0: Counting consecutive dibit==2
%            → If count >= 31, transition to State 1
%   State 1: Stay in this state as long as dibit==2
%            → If dibit==3, trigger detection and reset
%            → Else, reset

    % Persistent state and counter
    persistent state count_two
    if isempty(state)
        state = 0;
        count_two = 0;
    end

    % Default output
    preamble_detected = false;

    if start_of_symbol == 1
        switch state
            case 0
                if dibit == 2
                    count_two = count_two + 1;
                    if count_two >= 31
                        state = 1; % Start monitoring for dibit==3
                    end
                else
                    count_two = 0;
                end

            case 1
                if dibit == 2
                    % Stay in this state, continue accepting more 2s
                    % No change to count_two
                elseif dibit == 3
                    % Preamble matched
                    preamble_detected = true;
                    % Reset
                    state = 0;
                    count_two = 0;
                else
                    % Invalid sequence; reset
                    state = 0;
                    count_two = 0;
                end
        end
    end
end

== stateflow chart FULL_LINK/transmitter_with_phy/modulator_with_preamble_insertion/Preamble_inserter/Chart ==
  settings: executeAtInitialization=1
  state wait_start
    input_data_byte=0;
    select_data_preamble=1;
  state wait_byte_end
    input_data_byte=0;
    select_data_preamble=1;
  state send_start_of_data1
    input_data_byte=170;
    select_data_preamble=0;
  state send_stop_of_data2
    input_data_byte=170;
    select_data_preamble=0;
  state send_stop_of_data3
    input_data_byte=170;
    select_data_preamble=0;
  state send_start_of_data4
    input_data_byte=170;
    select_data_preamble=0;
  state send_start_of_data5
    input_data_byte=170;
    select_data_preamble=0;
  state send_stop_of_frame_delimiter1
    input_data_byte=171;
    select_data_preamble=0;
  note: [byte_end== 1 ]
  state send_stop_of_data7
    input_data_byte=170;
    select_data_preamble=0;
  state send_stop_of_data6
    input_data_byte=170;
    select_data_preamble=0;
  (default) -> wait_start
  wait_start -> wait_byte_end : [start==1]
  wait_byte_end -> send_start_of_data1 : [byte_end==1]
  send_stop_of_frame_delimiter1 -> wait_start : [byte_end==1]
  send_stop_of_data3 -> send_start_of_data4 : [byte_end==1]
  send_start_of_data1 -> send_stop_of_data2 : [byte_end==1]
  send_start_of_data4 -> send_start_of_data5 : [byte_end==1]
  send_stop_of_data2 -> send_stop_of_data3 : [byte_end==1]
  send_start_of_data5 -> send_stop_of_data6 : [byte_end==1]
  send_stop_of_data7 -> send_stop_of_frame_delimiter1
  send_stop_of_data6 -> send_stop_of_data7 : [byte_end==1]
  data: byte_end input; start input; input_data_byte output; select_data_preamble output

== matlab function FULL_LINK/transmitter_with_phy/modulator_with_preamble_insertion/Modulator_with_byte_input/MATLAB Function ==
  settings: fimath=fimath('RoundingMethod', 'Floor','OverflowAction', 'Wrap','ProductMode', 'FullPrecision', 'SumMode', 'FullPrecision')
  data: en input; dibit output; reset input; data_in input; byte_end output; bit_msb output; bit_lsb output
function [dibit, byte_end, bit_msb, bit_lsb] = dibit_extractor(en, reset, data_in)
% dibit_extractor  Extracts two-bit segments from an 8-bit input on enable pulses
%   en        : boolean enable signal (rising edge triggers output update)
%   reset     : boolean reset signal (synchronous reset of internal state)
%   data_in   : uint8 8-bit input data
%   dibit     : UFix_2_0 2-bit unsigned fixed-point output
%   byte_end  : real scalar; goes high every four dibits (i.e., end of byte)
%   bit_msb   : logical scalar; the most-significant bit of the dibit
%   bit_lsb   : logical scalar; the least-significant bit of the dibit

%#codegen

persistent count prev_en
if isempty(count)
    count   = uint8(3);   % cycle index (0 to 3)
    prev_en = 0;          % previous enable state
end

% Default outputs
byte_end = 0;
bit_msb  = false;
bit_lsb  = false;

% Synchronous reset
if reset
    count = uint8(0);
else
    % Detect rising edge of enable
    if en == 1 && prev_en == 0
        % Increment and wrap count
        count = mod(count + 1, 4);

        % Pulse byte_end when completing the fourth dibit
        if count == 1
            byte_end = 1;
        end
    end
end

prev_en = en;

% Determine starting bit position (0-based)
startBit = count * 2;

% Extract two bits (MATLAB bitget uses 1-based positions)
bit0 = bitget(data_in, startBit + 1);  % LSB of the dibit
bit1 = bitget(data_in, startBit + 2);  % MSB of the dibit

% Expose individual bits as Booleans
bit_lsb = logical(bit0);
bit_msb = logical(bit1);

% Assemble value (bit1 is MSB, bit0 is LSB)
value = uint8(bit1) * 2 + uint8(bit0);

% Create 2-bit unsigned fixed-point output
dibit = fi(value, 0, 2, 0);
end

== matlab function FULL_LINK/receiver_with_phy/demodulator_with_preamble_detector/MATLAB Function1 ==
  settings: fimath=fimath('RoundingMethod', 'Floor','OverflowAction', 'Wrap','ProductMode', 'FullPrecision', 'SumMode', 'FullPrecision')
  data: en input; data_out output; reset input; dibit input; byte_end output
function [data_out,byte_end] = byte_assembler(en, reset, dibit)
% byte_assembler  Assembles 8-bit data from four 2-bit segments
%   en        : boolean enable signal (rising edge triggers input sampling)
%   reset     : boolean reset signal (synchronous reset of internal state)
%   dibit     : ufix2 2-bit input
%   data_out  : uint8 8-bit output, valid after 4 dibits

%#codegen

persistent count temp_byte prev_en
if isempty(count)
    count = uint8(0);
    temp_byte = uint8(0);
    prev_en = 0;
    byte_end = 0;
end

% Synchronous reset
if reset
    count = uint8(1);
    temp_byte = uint8(0);
    byte_end = 0;
end

% Detect rising edge of enable
if en==1 && prev_en==0 && reset==0
    shift = bitshift(uint8(dibit), count * 2);  % Place dibit at the correct position
    mask = bitshift(uint8(3), count * 2);       % Create mask for clearing that position
    temp_byte = bitor(bitand(temp_byte, bitcmp(mask, 'uint8')), shift);

    % Increment count and wrap
    count = mod(count + 1, 4);
end
prev_en = en;

% Output the assembled byte only when 4 dibits have been collected
if count == 0 && reset==0
    data_out = temp_byte;
    byte_end = 1;
else
    data_out = uint8(0);
    byte_end = 0;
end
end
